simulink model "Generate_T_Matrix_VSC"  (R2024a)
settings: Solver=ode2  StartTime=0.0  StopTime=T_end  RelTol=1e-3  EnableMultiTasking=on
values from neighbouring files (symbols this model uses):
  Ts = 5e-6    (= 5e-06)    [Generate_T_Matrix.m]    (also in Test_T_Matrix.m)
undefined symbols (not defined in the file or in its folder): level
libraries: spsControlledVoltageSourceLib x4, powerlib_extras x3, spsThreePhaseVIMeasurementLib x3, spsGroundLib x3, spsSeriesRLCBranchLib x3, simulink_extras x2, spsabctodq0Lib x2, spsUniversalBridgeLib x1, spsdq0toabcLib x1, spsThreePhaseSeriesRLCBranchLib x1, spsVoltageMeasurementLib x1, spspowerguiLib x1
settings Model: Creator=GAO_CX  LastModifiedBy=GAO_CX
settings DataIOCC: SaveOutput=off  SignalLogging=off  DSMLogging=off  SaveTime=off  ReturnWorkspaceOutputs=off

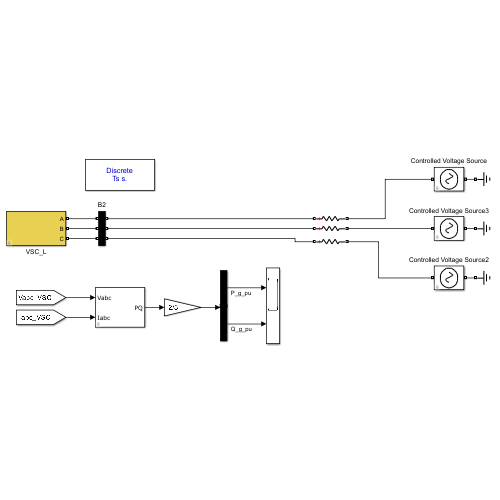
[thumbnail: Simulink's stored preview of the top-level diagram]
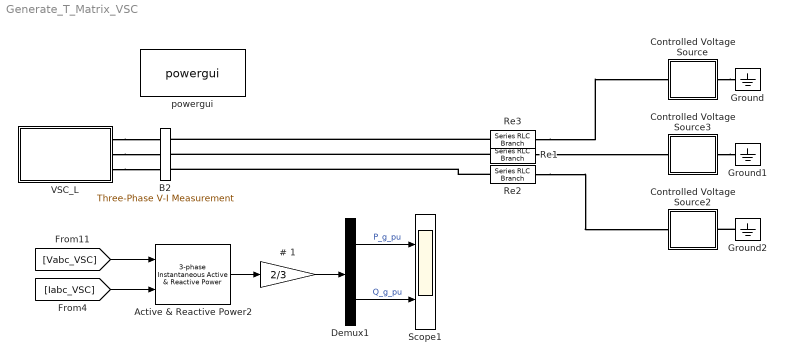
== system Generate_T_Matrix_VSC ==
  # 1 : Gain  Gain=2/3  SaturateOnIntegerOverflow=on  OutDataTypeStr=Inherit: Same as input  ParamDataTypeStr=Inherit: Same as input
  Active & Reactive Power2 : powerlib_extras/Measurements/3-phase  Instantaneous  Active & Reactive Power
  B2 : spsThreePhaseVIMeasurementLib/Three-Phase V-I Measurement  VoltageMeasurement=phase-to-ground  SetLabelV=on  LabelV=Vabc_VSC  Vpu=on  VpuLL=off  CurrentMeasurement=yes  SetLabelI=on  LabelI=Iabc_VSC  Ipu=on  Pbase=1e6  Vbase=50  OutputType=Complex  PhasorSimulation=off  PSBequivalent=0
  Controlled Voltage Source : Subsystem  mask{amp=300, fac=60, ramp=0.05, ini_phase=0}
      mask prompts: amp "Peak voltage (V)"; fac "Frequency (Hz)"; ramp "Ramp up time (s)"; ini_phase "Initial phase (deg)"
      mask DialogControl ParameterGroupVar Prompt: 参数
      mask Display: plot(-50,-35,50,50-15,[0,9,18,24,29,30,29,24,18,9,0,-9,-18,-24,-29,-30,-29,-24,-18,-9,0],[30,29,24,18,9,0,-9,-18,-24,-29,-30,-29,-24,-18,-9,0,9,18,24,29,30],[0,9,18,24,29,30,29,24,18,9,0,-9,-18,-24,-29,-30,-29,-24,-18,-9,0]./-2.4,[1 2 3 4 5 6 7 8 9 10 11 12 13 14 15 16 17 18 19 20 21].*1.5-15);
  Controlled Voltage Source2 : Subsystem  mask{amp=500, fac=50, ramp=0.05, ini_phase=30}
      mask prompts: amp "Peak voltage (V)"; fac "Frequency (Hz)"; ramp "Ramp up time (s)"; ini_phase "Initial phase (deg)"
      mask DialogControl ParameterGroupVar Prompt: 参数
      mask Display: plot(-50,-35,50,50-15,[0,9,18,24,29,30,29,24,18,9,0,-9,-18,-24,-29,-30,-29,-24,-18,-9,0],[30,29,24,18,9,0,-9,-18,-24,-29,-30,-29,-24,-18,-9,0,9,18,24,29,30],[0,9,18,24,29,30,29,24,18,9,0,-9,-18,-24,-29,-30,-29,-24,-18,-9,0]./-2.4,[1 2 3 4 5 6 7 8 9 10 11 12 13 14 15 16 17 18 19 20 21].*1.5-15);
  Controlled Voltage Source3 : Subsystem  mask{amp=400, fac=100, ramp=0.05, ini_phase=120}
      mask prompts: amp "Peak voltage (V)"; fac "Frequency (Hz)"; ramp "Ramp up time (s)"; ini_phase "Initial phase (deg)"
      mask DialogControl ParameterGroupVar Prompt: 参数
      mask Display: plot(-50,-35,50,50-15,[0,9,18,24,29,30,29,24,18,9,0,-9,-18,-24,-29,-30,-29,-24,-18,-9,0],[30,29,24,18,9,0,-9,-18,-24,-29,-30,-29,-24,-18,-9,0,9,18,24,29,30],[0,9,18,24,29,30,29,24,18,9,0,-9,-18,-24,-29,-30,-29,-24,-18,-9,0]./-2.4,[1 2 3 4 5 6 7 8 9 10 11 12 13 14 15 16 17 18 19 20 21].*1.5-15);
  Demux1 : Demux  Outputs=2
      settings: DisplayOption=none
  Ground : spsGroundLib/Ground  LConnTagsString=a
  Ground1 : spsGroundLib/Ground  LConnTagsString=a
  Ground2 : spsGroundLib/Ground  LConnTagsString=a
  Re1 : spsSeriesRLCBranchLib/Series RLC Branch  LConnTagsString=__new0  RConnTagsString=__new0  BranchType=R  Resistance=0.3  Inductance=0.003  SetiL0=off  InitialCurrent=0  Capacitance=1e-6  Setx0=off  InitialVoltage=0  Measurements=None
  Re2 : spsSeriesRLCBranchLib/Series RLC Branch  LConnTagsString=__new0  RConnTagsString=__new0  BranchType=R  Resistance=0.5  Inductance=0.003  SetiL0=off  InitialCurrent=0  Capacitance=1e-6  Setx0=off  InitialVoltage=0  Measurements=None
  Re3 : spsSeriesRLCBranchLib/Series RLC Branch  LConnTagsString=__new0  RConnTagsString=__new0  BranchType=R  Resistance=0.01  Inductance=0.003  SetiL0=off  InitialCurrent=0  Capacitance=1e-6  Setx0=off  InitialVoltage=0  Measurements=None
  Scope1 : Scope  NumInputPorts=2
  VSC_L : Subsystem  mask{P_rated=1e6, Vac_rated=380, Vdc_rated=1200, f_rated=50, Pref=1.0, Qref=0, Rf1_pu=1e-3, Lf1_pu=0.5, KP_PLL=5, KI_PLL=100, KP_ig=5, KI_ig=10, KP_P=0.2, KI_P=100}
      mask prompts: P_rated "Rated Power (W)"; Vac_rated "Rated AC voltage (V)"; Vdc_rated "Rated DC voltage (V)"; f_rated "Rated grid frequency"; Rf1_pu "Filter resistor Rf1 (pu)"; Lf1_pu "Filter inductor Lf1 (pu)"; KP_PLL "P of PLL"; KI_PLL "I of PLL"; KP_ig "P of current PI  controller"; KI_ig "I of current PI  controller"; KP_P "P of power PI  controller"; KI_P "I of power PI  controller"
      mask init:
      | Z_rated=Vac_rated*Vac_rated/P_rated;
      | % transformer to pu
      | wg_rated=2*pi*f_rated;
      | Lg_rated=Z_rated/wg_rated;
      | Cg_rated=1/Z_rated/wg_rated;
      | 
      | Rf1=Z_rated*Rf1_pu;
      | Lf1=Lg_rated*Lf1_pu;
      mask DialogControl Basic_Parameters Prompt: Basic Parameters
      mask DialogControl GSC Prompt: GSC Parameters
  powergui : spspowerguiLib/powergui  SimulationMode=Discrete  SampleTime=Ts  frequency=50  Iterations=50  frequencyindice=0  Pbase=100e6  ErrMax=1e-4  UnitsV=kV  UnitsW=MW  buscounter=6  FunctionMessages=off  echomessages=off  EnableUseOfTLC=off  CurrentSourceSwitches=off  DisableSnubberDevices=off  DisableRonSwitches=off  DisableVfSwitches=off  DisplayEquations=off  AutomaticDiscreteSolvers=off  SolverType=Tustin  Interpol=off  ExternalGateDelay=off  methode=off  Ts=0  x0status=blocks  SPID=off  SwTol=0  HookPort=off  NonlinearTolerance=1e-4  nMaxIteration=100  ContinueOnMaxIteration=off  RestoreLinks=warning  ResistiveCurrentMeasurement=off  Frange=[0:2:500]  Ylog=off  Xlog=on  ShowGrid=off  save=off  variable=ZData  structure=0  ZoomFFT=on  StartTime=0.0  cycles=1  DisplayStyle=1  fundamental=60  FreqAxis=off  MaxFrequency=1000  frequencyindicesteady=1  RmsSteady=1  display=off
  wires:
  [Vabc_VSC] -> Active & Reactive Power2/1
  Demux1/1 -> Scope1/1  "P_g_pu"
  Demux1/2 -> Scope1/2  "Q_g_pu"
  [Iabc_VSC] -> Active & Reactive Power2/2
  Active & Reactive Power2/1 -> # 1/1
  # 1/1 -> Demux1/1
  connections:
  Controlled Voltage Source3/LConn1 -- Ground1/LConn1
  Re3/LConn1 -- B2/RConn1
  VSC_L/LConn2 -- B2/LConn2
  Re2/RConn1 -- Controlled Voltage Source2/RConn1
  Re2/LConn1 -- B2/RConn3
  Ground2/LConn1 -- Controlled Voltage Source2/LConn1
  VSC_L/LConn1 -- B2/LConn1
  Re3/RConn1 -- Controlled Voltage Source/RConn1
  Controlled Voltage Source/LConn1 -- Ground/LConn1
  Re1/LConn1 -- B2/RConn2
  VSC_L/LConn3 -- B2/LConn3
  Re1/RConn1 -- Controlled Voltage Source3/RConn1

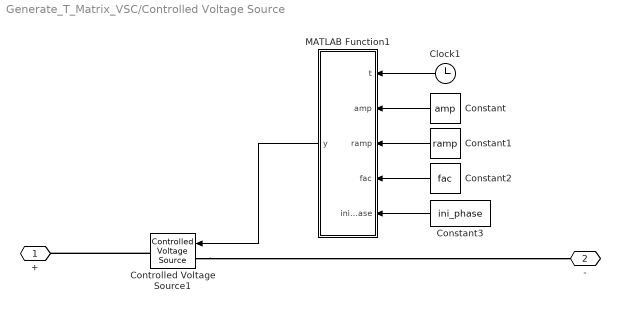
== system Generate_T_Matrix_VSC/Controlled Voltage Source ==
  Clock1 : Clock
  Constant : Constant  Value=amp
  Constant1 : Constant  Value=ramp
  Constant2 : Constant  Value=fac
  Constant3 : Constant  Value=ini_phase
  Controlled Voltage Source1 : spsControlledVoltageSourceLib/Controlled Voltage Source  Initialize=off  Source_Type=DC  Amplitude=0  Phase=0  Frequency=0  Measurements=None
  MATLAB Function1 : MATLAB Function  TreatAsAtomicUnit=on
  + : PMIOPort  Side=Right
  - : PMIOPort  Port=2  Side=Left
  wires:
  Constant/1 -> MATLAB Function1/2(amp)
  Clock1/1 -> MATLAB Function1/1(t)
  Constant2/1 -> MATLAB Function1/4(fac)
  Constant1/1 -> MATLAB Function1/3(ramp)
  Constant3/1 -> MATLAB Function1/5(ini_phase)
  MATLAB Function1/1(y) -> Controlled Voltage Source1/1
  connections:
  Controlled Voltage Source1/RConn1 -- +/RConn1
  Controlled Voltage Source1/LConn1 -- -/RConn1

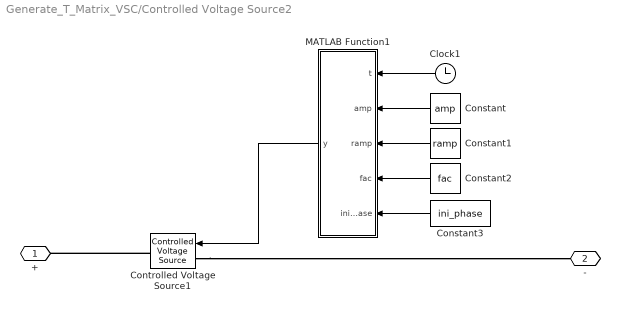
== system Generate_T_Matrix_VSC/Controlled Voltage Source2 ==
  Clock1 : Clock
  Constant : Constant  Value=amp
  Constant1 : Constant  Value=ramp
  Constant2 : Constant  Value=fac
  Constant3 : Constant  Value=ini_phase
  Controlled Voltage Source1 : spsControlledVoltageSourceLib/Controlled Voltage Source  Initialize=off  Source_Type=DC  Amplitude=0  Phase=0  Frequency=0  Measurements=None
  MATLAB Function1 : MATLAB Function  TreatAsAtomicUnit=on
  + : PMIOPort  Side=Right
  - : PMIOPort  Port=2  Side=Left
  wires:
  Constant/1 -> MATLAB Function1/2(amp)
  Clock1/1 -> MATLAB Function1/1(t)
  Constant2/1 -> MATLAB Function1/4(fac)
  Constant1/1 -> MATLAB Function1/3(ramp)
  Constant3/1 -> MATLAB Function1/5(ini_phase)
  MATLAB Function1/1(y) -> Controlled Voltage Source1/1
  connections:
  Controlled Voltage Source1/RConn1 -- +/RConn1
  Controlled Voltage Source1/LConn1 -- -/RConn1

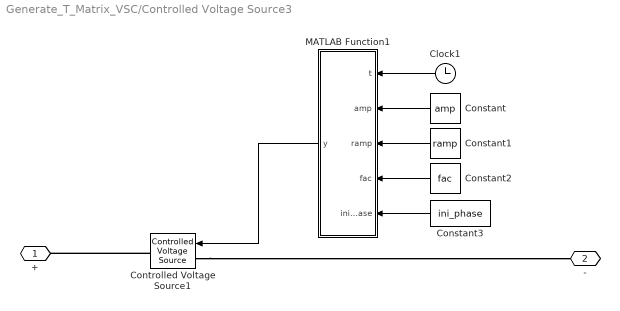
== system Generate_T_Matrix_VSC/Controlled Voltage Source3 ==
  Clock1 : Clock
  Constant : Constant  Value=amp
  Constant1 : Constant  Value=ramp
  Constant2 : Constant  Value=fac
  Constant3 : Constant  Value=ini_phase
  Controlled Voltage Source1 : spsControlledVoltageSourceLib/Controlled Voltage Source  Initialize=off  Source_Type=DC  Amplitude=0  Phase=0  Frequency=0  Measurements=None
  MATLAB Function1 : MATLAB Function  TreatAsAtomicUnit=on
  + : PMIOPort  Side=Right
  - : PMIOPort  Port=2  Side=Left
  wires:
  Constant/1 -> MATLAB Function1/2(amp)
  Clock1/1 -> MATLAB Function1/1(t)
  Constant2/1 -> MATLAB Function1/4(fac)
  Constant1/1 -> MATLAB Function1/3(ramp)
  Constant3/1 -> MATLAB Function1/5(ini_phase)
  MATLAB Function1/1(y) -> Controlled Voltage Source1/1
  connections:
  Controlled Voltage Source1/RConn1 -- +/RConn1
  Controlled Voltage Source1/LConn1 -- -/RConn1

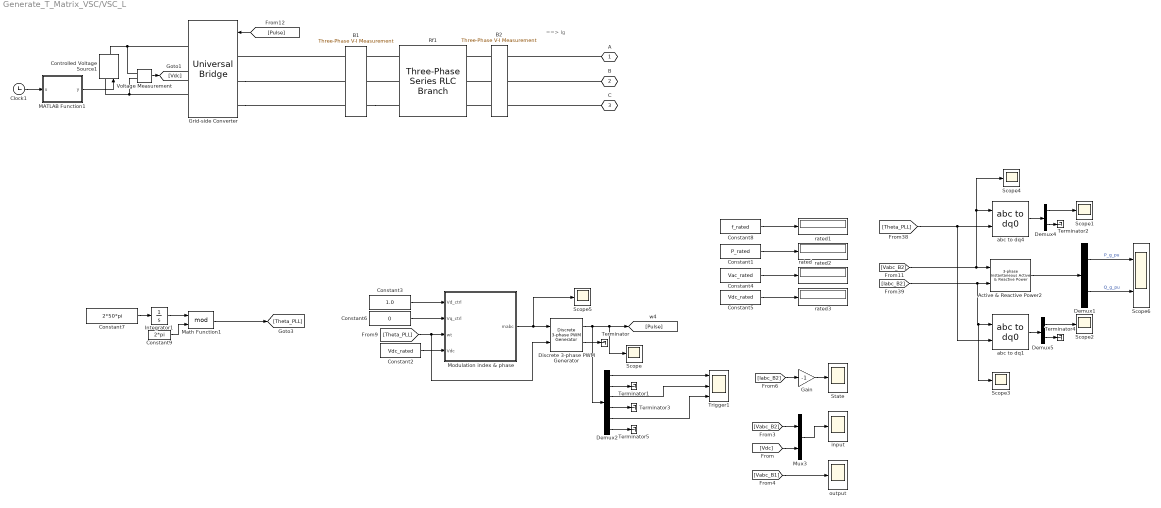
== system Generate_T_Matrix_VSC/VSC_L ==
  note: ==> Ig
  Active & Reactive Power2 : powerlib_extras/Measurements/3-phase  Instantaneous  Active & Reactive Power
  B1 : spsThreePhaseVIMeasurementLib/Three-Phase V-I Measurement  VoltageMeasurement=phase-to-ground  SetLabelV=on  LabelV=Vabc_B1  Vpu=off  VpuLL=off  CurrentMeasurement=no  SetLabelI=off  LabelI=Iabc_B2  Ipu=off  Pbase=P_rated  Vbase=Vac_rated  OutputType=Complex  PhasorSimulation=off  PSBequivalent=0
  B2 : spsThreePhaseVIMeasurementLib/Three-Phase V-I Measurement  VoltageMeasurement=phase-to-ground  SetLabelV=on  LabelV=Vabc_B2  Vpu=off  VpuLL=off  CurrentMeasurement=yes  SetLabelI=on  LabelI=Iabc_B2  Ipu=off  Pbase=P_rated  Vbase=Vac_rated  OutputType=Complex  PhasorSimulation=off  PSBequivalent=0
  Clock1 : Clock
  Constant1 : Constant  Value=P_rated
  Constant2 : Constant  Value=Vdc_rated
  Constant3 : Constant  Value=1.0
  Constant4 : Constant  Value=Vac_rated
  Constant5 : Constant  Value=Vdc_rated
  Constant6 : Constant  Value=0
  Constant7 : Constant  Value=2*50*pi
  Constant8 : Constant  Value=f_rated
  Constant9 : Constant  Value=2*pi
  Controlled Voltage Source1 : spsControlledVoltageSourceLib/Controlled Voltage Source  Initialize=on  Source_Type=DC  Amplitude=0  Phase=0  Frequency=0  Measurements=None
  Demux1 : Demux  Outputs=2
      settings: DisplayOption=none
  Demux2 : Demux  Outputs=6
      settings: DisplayOption=none
  Demux4 : Demux  Outputs=[2 1]
      settings: DisplayOption=none
  Demux5 : Demux  Outputs=[2 1]
      settings: DisplayOption=none
  Discrete 3-phase PWM Generator : powerlib_extras/Discrete  Control Blocks/Discrete 3-phase PWM Generator  ModulatorType=2-level  ModulatorMode=Synchronized  nF=100  Fc=2700  ModulatingSignals=off  m=0.2  Freq=60  Phase=0  Ts=Ts
  Gain : Gain  Gain=-1
  Grid-side Converter : spsUniversalBridgeLib/Universal Bridge  Arms=3  SnubberResistance=1e6  SnubberCapacitance=inf  Device=IGBT / Diodes  Ron=0.01  Lon=0  ForwardVoltages="[  0  0  ]"  ForwardVoltage=0  GTOparameters=[ 10e-6 , 20e-6 ]  IGBTparameters=[0 , 0]  Measurements=None  Measurements_2=None  converterType=Rectifier
  Integrator1 : Integrator
  MATLAB Function1 : MATLAB Function  TreatAsAtomicUnit=on
  Math Function1 : Math  Operator=mod
  "Modulation index & phase " : Subsystem
  Mux3 : Mux  Inputs=2
  Rf1 : spsThreePhaseSeriesRLCBranchLib/Three-Phase Series RLC Branch  LConnTagsString=A|B|C  RConnTagsString=A|B|C  BranchType=RL  Resistance=Rf1  Inductance=Lf1  Capacitance=1.0  Measurements=None
  Scope{,1..5} (6 alike) : Scope
  Scope6 : Scope  NumInputPorts=2
  State : Scope
  Terminator{,1..5} (6 alike) : Terminator
  Trigger1 : Scope  NumInputPorts=3
  Voltage Measurement : spsVoltageMeasurementLib/Voltage Measurement  PhasorSimulation=off  OutputType=Complex  PSBequivalent=0
  abc to dq1 : spsabctodq0Lib/abc to dq0  Alignment=90 degrees behind phase A axis
  abc to dq4 : spsabctodq0Lib/abc to dq0  Alignment=90 degrees behind phase A axis
  input : Scope
  output : Scope
  rated{,1..3} (4 alike) : Display
  A : PMIOPort  Tag=PMCPort  Side=Left
  B : PMIOPort  Tag=PMCPort  Port=2  Side=Left
  C : PMIOPort  Tag=PMCPort  Port=3  Side=Left
  wires:
  [Theta_PLL] -> Discrete 3-phase PWM Generator/2, "Modulation index & phase "/3(wt)
  Constant2/1 -> "Modulation index & phase "/4(Vdc)
  Constant3/1 -> "Modulation index & phase "/1(Vd_ctrl)
  Constant6/1 -> "Modulation index & phase "/2(Vq_ctrl)
  [Pulse] -> Grid-side Converter/1
  abc to dq1/1 -> Demux5/1
  Constant5/1 -> rated3/1
  Constant4/1 -> rated/1
  Demux5/1 -> Scope2/1
  [Iabc_B2] -> Scope3/1, abc to dq1/1, Active & Reactive Power2/2
  Demux1/1 -> Scope6/1  "P_g_pu"
  Demux4/1 -> Scope1/1
  [Vabc_B2] -> Scope4/1, abc to dq4/1, Active & Reactive Power2/1
  Constant1/1 -> rated2/1
  [Theta_PLL] -> abc to dq1/2, abc to dq4/2
  Constant8/1 -> rated1/1
  abc to dq4/1 -> Demux4/1
  Active & Reactive Power2/1 -> Demux1/1
  Demux5/2 -> Terminator4/1
  Demux1/2 -> Scope6/2  "Q_g_pu"
  Demux4/2 -> Terminator2/1
  Discrete 3-phase PWM Generator/2 -> Terminator/1
  Discrete 3-phase PWM Generator/1 -> Demux2/1, Scope/1, [Pulse]
  "Modulation index & phase "/1(mabc) -> Scope5/1, Discrete 3-phase PWM Generator/1
  Demux2/1 -> Trigger1/1
  Demux2/2 -> Terminator1/1
  Demux2/3 -> Trigger1/2
  Demux2/5 -> Trigger1/3
  Demux2/4 -> Terminator3/1
  Demux2/6 -> Terminator5/1
  [Iabc_B2] -> Gain/1
  [Vabc_B1] -> output/1
  Clock1/1 -> MATLAB Function1/1(u)
  MATLAB Function1/1(y) -> Controlled Voltage Source1/1
  Math Function1/1 -> [Theta_PLL]
  Integrator1/1 -> Math Function1/1
  Constant7/1 -> Integrator1/1
  Constant9/1 -> Math Function1/2
  Voltage Measurement/1 -> [Vdc]
  [Vabc_B2] -> Mux3/1
  [Vdc] -> Mux3/2
  Mux3/1 -> input/1
  Gain/1 -> State/1
  connections:
  C/RConn1 -- B2/RConn3
  B/RConn1 -- B2/RConn2
  A/RConn1 -- B2/RConn1
  Grid-side Converter/RConn2 -- Voltage Measurement/LConn2 -- Controlled Voltage Source1/LConn1
  Grid-side Converter/RConn1 -- Voltage Measurement/LConn1 -- Controlled Voltage Source1/RConn1
  B2/LConn1 -- Rf1/LConn1
  B2/LConn2 -- Rf1/LConn2
  B2/LConn3 -- Rf1/LConn3
  Rf1/RConn2 -- B1/RConn2
  Rf1/RConn1 -- B1/RConn1
  B1/RConn3 -- Rf1/RConn3
  B1/LConn1 -- Grid-side Converter/LConn1
  Grid-side Converter/LConn2 -- B1/LConn2
  Grid-side Converter/LConn3 -- B1/LConn3

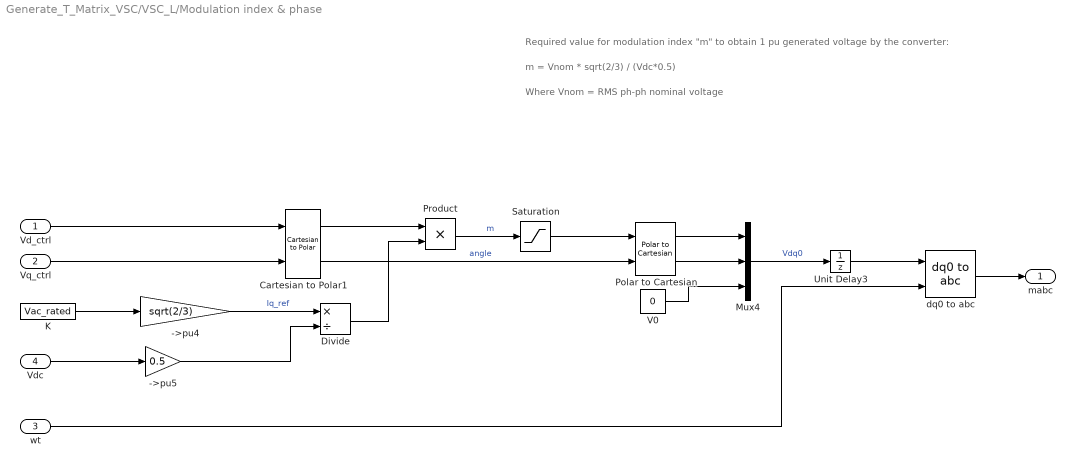
== system Generate_T_Matrix_VSC/VSC_L/Modulation index & phase  ==
  note: Where Vnom = RMS ph-ph nominal voltage
  note: m = Vnom * sqrt(2/3) / (Vdc*0.5)
  note: Required value for modulation index "m" to obtain 1 pu generated voltage by the converter:
  Vd_ctrl : Inport
  Vq_ctrl : Inport  Port=2
  wt : Inport  Port=3
  Vdc : Inport  Port=4
  ->pu4 : Gain  Gain=sqrt(2/3)
  ->pu5 : Gain  Gain=0.5
  Cartesian to Polar1 : simulink_extras/Transformations/Cartesian to Polar
  Divide : Product  Inputs=*/
  K : Constant  Value=Vac_rated
  Mux4 : Mux  Inputs=3
  Polar to Cartesian : simulink_extras/Transformations/Polar to Cartesian
  Product : Product
  Saturation : Saturate  UpperLimit=1  LowerLimit=0
  Unit Delay3 : UnitDelay  SampleTime=-1
  V0 : Constant  Value=0
  dq0 to abc : spsdq0toabcLib/dq0 to abc  Alignment=90 degrees behind phase A axis
  mabc : Outport
  wires:
  Cartesian to Polar1/1 -> Product/1
  Mux4/1 -> Unit Delay3/1  "Vdq0"
  Product/1 -> Saturation/1  "m"
  V0/1 -> Mux4/3
  Cartesian to Polar1/2 -> Polar to Cartesian/2  "angle"
  Vdc/1 -> ->pu5/1
  dq0 to abc/1 -> mabc/1
  K/1 -> ->pu4/1
  Vq_ctrl/1 -> Cartesian to Polar1/2
  wt/1 -> dq0 to abc/2
  Vd_ctrl/1 -> Cartesian to Polar1/1
  ->pu5/1 -> Divide/2
  ->pu4/1 -> Divide/1  "Iq_ref"
  Divide/1 -> Product/2
  Polar to Cartesian/1 -> Mux4/1
  Polar to Cartesian/2 -> Mux4/2
  Unit Delay3/1 -> dq0 to abc/1
  Saturation/1 -> Polar to Cartesian/1

== matlab function Generate_T_Matrix_VSC/Controlled Voltage Source/MATLAB Function1 ==
  data: t input; y output; amp input; ramp input; fac input; ini_phase input
function y = fcn(t,amp,ramp,fac,ini_phase)
   y=min(t*(amp/ramp),amp)*sin(2*pi*fac*t+ini_phase/180*pi);

== matlab function Generate_T_Matrix_VSC/Controlled Voltage Source2/MATLAB Function1 ==
  data: t input; y output; amp input; ramp input; fac input; ini_phase input
function y = fcn(t,amp,ramp,fac,ini_phase)
   y=min(t*(amp/ramp),amp)*sin(2*pi*fac*t+ini_phase/180*pi);

== matlab function Generate_T_Matrix_VSC/VSC_L/MATLAB Function1 ==
  data: u input; y output
function y = fcn(u)
   y=1200+min(u*(10/0.05),10)*sin(2*pi*50*u);

== matlab function Generate_T_Matrix_VSC/Controlled Voltage Source3/MATLAB Function1 ==
  data: t input; y output; amp input; ramp input; fac input; ini_phase input
function y = fcn(t,amp,ramp,fac,ini_phase)
   y=min(t*(amp/ramp),amp)*sin(2*pi*fac*t+ini_phase/180*pi);
